simulink subsystem "CO2_dissociation_inv"  (R2020b)
settings: Solver=VariableStepAuto  StartTime=0.0  StopTime=10.0  RelTol=1e-3
settings Model: Creator=RH  LastModifiedBy=Marco

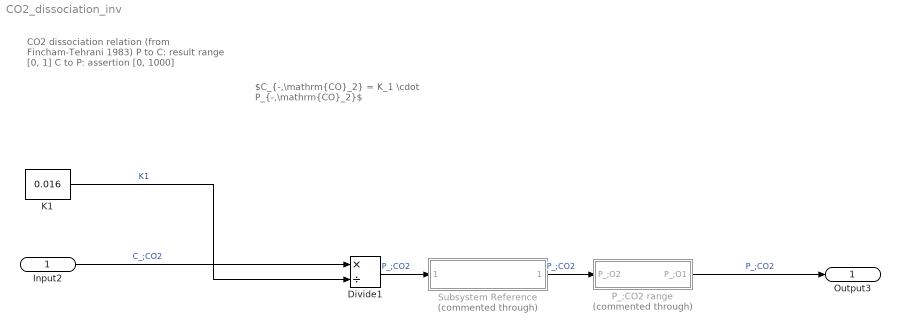
== system CO2_dissociation_inv ==
  note: $C_{-,\mathrm{CO}_2} = K_1 \cdot P_{-,\mathrm{CO}_2}$
  note: CO2 dissociation relation
      | (from Fincham-Tehrani 1983)
      |
      | P to C: result range [0, 1]
      | C to P: assertion [0, 1000]
  Input2 : Inport  Unit=1
  Divide1 : Product  Inputs=*/
  K1 : Constant  Value=0.016
  P_;CO2 range : Subsystem  Commented=through
  Subsystem Reference : Subsystem  Commented=through  ReferencedSubsystem=saturation_range
  Output3 : Outport  Unit=mmHg
  wires:
  Input2/1 -> Divide1/1  "C_;CO2"
  K1/1 -> Divide1/2  "K1"
  Divide1/1 -> Subsystem Reference/1  "P_;CO2"
  Subsystem Reference/1 -> P_;CO2 range/1(P_;O2)  "P_;CO2"
  P_;CO2 range/1(P_;O1) -> Output3/1  "P_;CO2"

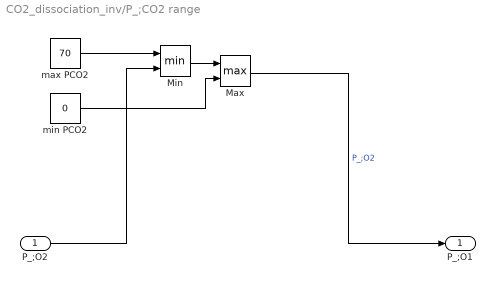
== system CO2_dissociation_inv/P_;CO2 range ==
  P_;O2 : Inport
  Max : MinMax  Function=max  Inputs=2
  Min : MinMax  Inputs=2
  max PCO2 : Constant  Value=70
  min PCO2 : Constant  Value=0
  P_;O1 : Outport
  wires:
  P_;O2/1 -> Min/2
  Min/1 -> Max/1
  max PCO2/1 -> Min/1
  min PCO2/1 -> Max/2
  Max/1 -> P_;O1/1  "P_;O2"
